simulink model "feedback_harness"  (R2013a)
settings: Solver=ode45  StartTime=0.0  StopTime=10  RelTol=1e-3
settings Model: ModifiedByFormat=The MathWorks Inc.  Creator=The MathWorks Inc.  LastModifiedBy=The MathWorks Inc.
settings DataIOCC: SaveOutput=off  SaveTime=off
settings OptimizationCC: ExpressionDepthLimit=2147483647  LifeSpan=1
settings DebuggingCC: FcnCallInpInsideContextMsg=EnableAllAsWarning
settings GRTTargetCC: CombineOutputUpdateFcns=off  GRTInterface=on

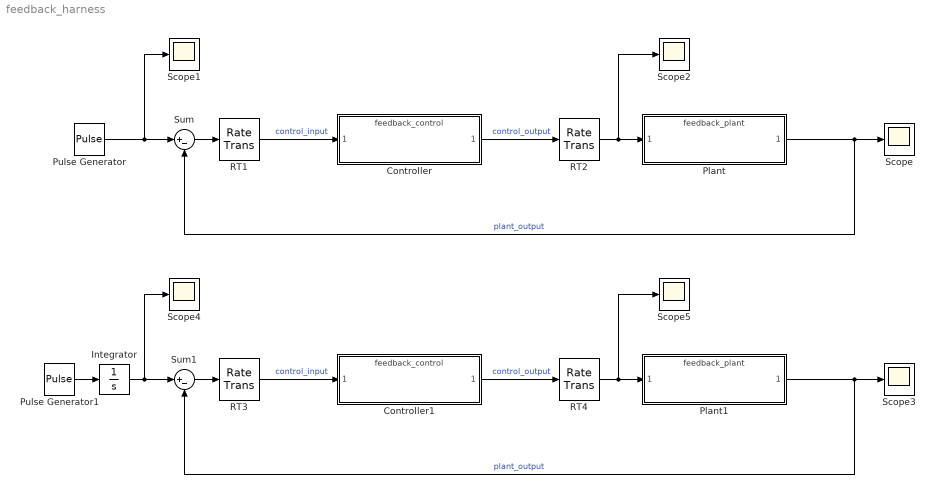
== system feedback_harness ==
  Controller : ModelReference  ModelNameDialog=feedback_control  SimulationMode=Normal  ModelReferenceVersion=1.41  CopyOfModelName=feedback_control  DefaultDataLogging=on
  Controller1 : ModelReference  ModelNameDialog=feedback_control  SimulationMode=Normal  ModelReferenceVersion=1.41  CopyOfModelName=feedback_control  DefaultDataLogging=on
  Integrator : Integrator
  Plant : ModelReference  ModelNameDialog=feedback_plant  SimulationMode=Normal  ModelReferenceVersion=1.23  CopyOfModelName=feedback_plant  DefaultDataLogging=on
  Plant1 : ModelReference  ModelNameDialog=feedback_plant  SimulationMode=Normal  ModelReferenceVersion=1.23  CopyOfModelName=feedback_plant  DefaultDataLogging=on
  Pulse Generator : DiscretePulseGenerator  PulseType=Time based  Period=4  PulseWidth=50
  Pulse Generator1 : DiscretePulseGenerator  PulseType=Time based  Period=4  PulseWidth=50
  RT{1..4} (4 alike) : RateTransition
  Scope{,1..5} (6 alike) : Scope
      Scope settings: TimeRange=1  YMin=0  YMax=1.4  SaveName=saida
      Scope1 settings: SaveName=entrada
      Scope2 settings: SaveName=controle
      Scope3 settings: TimeRange=1  YMin=0  YMax=1.4  SaveName=saida1
      Scope4 settings: SaveName=entrada1
      Scope5 settings: SaveName=controle1
  Sum : Sum  Inputs=|+-
  Sum1 : Sum  Inputs=|+-
  wires:
  Sum/1 -> RT1/1
  Controller/1 -> RT2/1  "control_output"
  Plant/1 -> Scope/1, Sum/2  "plant_output"
  RT1/1 -> Controller/1  "control_input"
  RT2/1 -> Scope2/1, Plant/1
  Pulse Generator/1 -> Scope1/1, Sum/1
  Sum1/1 -> RT3/1
  Controller1/1 -> RT4/1  "control_output"
  Plant1/1 -> Scope3/1, Sum1/2  "plant_output"
  RT3/1 -> Controller1/1  "control_input"
  RT4/1 -> Scope5/1, Plant1/1
  Pulse Generator1/1 -> Integrator/1
  Integrator/1 -> Scope4/1, Sum1/1
